simulink model "fromFileTest"  (R2024b)
settings: Solver=VariableStepAuto  StartTime=0.0  StopTime=10.0  MaxStep=1e-4  RelTol=1e-3
InitFcn:
  | % Working Directory
  | currDir = pwd;
  | % Parent Directory
  | cd('../PathGeneration/')
  | % Load Coeffs
  | run('pathGen_3D_proj.m')
  | % % Go back to cwd
  | % cd(currDir)
undefined symbols (not defined in the file or in its folder): coeffx, coeffy, coeffz
settings Model: Creator=Thoma  LastModifiedBy=Thoma

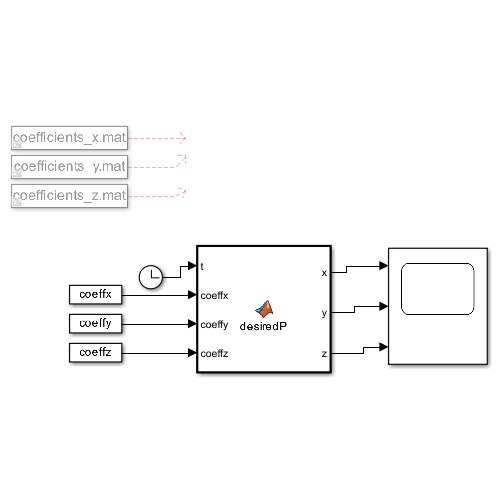
[thumbnail: Simulink's stored preview of the top-level diagram]
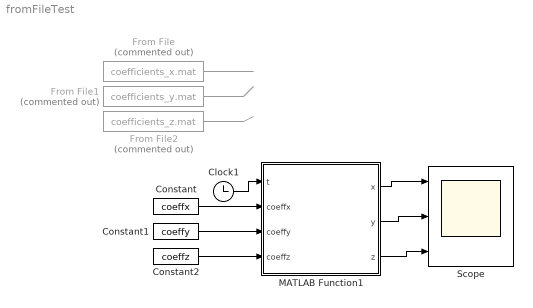
== system fromFileTest ==
  Clock1 : Clock
  Constant : Constant  Value=coeffx
  Constant1 : Constant  Value=coeffy
  Constant2 : Constant  Value=coeffz
  From File : FromFile  Commented=on  FileName=coefficients_x.mat  SampleTime=0
  From File1 : FromFile  Commented=on  FileName=coefficients_y.mat  SampleTime=0
  From File2 : FromFile  Commented=on  FileName=coefficients_z.mat  SampleTime=0
  MATLAB Function1 : MATLAB Function  TreatAsAtomicUnit=on
  Scope : Scope  NumInputPorts=3
  wires:
  From File/1 -> ?
  From File1/1 -> ?
  From File2/1 -> ?
  Clock1/1 -> MATLAB Function1/1(t)
  MATLAB Function1/1(x) -> Scope/1
  MATLAB Function1/2(y) -> Scope/2
  MATLAB Function1/3(z) -> Scope/3
  Constant/1 -> MATLAB Function1/2(coeffx)
  Constant1/1 -> MATLAB Function1/3(coeffy)
  Constant2/1 -> MATLAB Function1/4(coeffz)

== matlab function fromFileTest/MATLAB Function1 ==
  data: x output; t input; y output; z output; coeffx input; coeffy input; coeffz input
function [x,y,z] = desiredP(t, coeffx, coeffy, coeffz)
    
 %    coeffx = [2.0000
 %         0
 %         0
 %    0.1600
 %   -0.1600
 %    1.4400
 %    1.5200
 %   -1.2000
 %    0.2400
 %    2.0800
 %    0.5600
 %   -0.7200
 %    0.1600
 %   99.2800
 % -113.9200
 %   48.9600
 %   -9.2000
 %    0.6400];
 % 
 %    coeffy = [0.5000
 %         0
 %         0
 %   -3.3000
 %    2.3000
 %    6.3000
 %  -15.1000
 %   10.5000
 %   -2.2000
 %  -24.9000
 %   31.7000
 %  -12.9000
 %    1.7000
 %  218.1000
 % -246.4000
 %  103.2000
 %  -19.0000
 %    1.3000];
 % 
 %    coeffz = [1.6000
 %         0
 %         0
 %    0.2800
 %   -0.2800
 %    0.6200
 %    2.6600
 %   -2.1000
 %    0.4200
 %    1.7400
 %    0.9800
 %   -1.2600
 %    0.2800
 %  171.8400
 % -199.3600
 %   85.6800
 %  -16.1000
 %    1.1200];

    %%% From MAP Model %%%
    % A=0.05;
    % y=0.2+A*sin(2*t); % orig x
    % z=0.4+A*sin(2*t); % orig y
    % x=-0.205+A*sin(2*t); % orig z
    %%% From MAP Model %%%

    %%% Constant Test %%%
    x = 2.0; % [m]
    y = 0.5; % [m]
    z = 1.6; % [m]
    %%% Constant Test %%%

    %%% Hard code test from 3D path gen %%%
    % x = 0; y = 0; z = 0;
    tIntervals = [0 1 2 3 4]; % [sec] test hard code from 3Dpath

    if t <= tIntervals(2)
        x = F4(t)*coeffx(1:5);
        y = F4(t)*coeffy(1:5);
        z = F4(t)*coeffz(1:5);
    elseif t <= tIntervals(3)
        x = F3(t)*coeffx(6:9);
        y = F3(t)*coeffy(6:9);
        z = F3(t)*coeffz(6:9);
    elseif t <= tIntervals(4)
        x = F3(t)*coeffx(10:13);
        y = F3(t)*coeffy(10:13);
        z = F3(t)*coeffz(10:13);
    elseif t <= tIntervals(5)
        x = F4(t)*coeffx(14:18);
        y = F4(t)*coeffy(14:18);
        z = F4(t)*coeffz(14:18);
    % else
    %     y = 2.0; % [m]
    %     x = 0.5; % [m]
    %     z = 1.6; % [m]
    end

    function [out] = F4(t) 
        out =   [1   t    t.^2    t.^3     t.^4];
    end
    function [out] = F3(t) 
        out =   [1   t    t.^2    t.^3];
    end
    %%% Hard code test from 3D path gen %%%

end
